simulink model "LPDs_single_agent_tech"  (R2023b)
settings: Solver=VariableStepAuto  StartTime=0.0  StopTime=24  FixedStep=0.005  RelTol=1e-6
undefined symbols (not defined in the file): battery_capacity_state_lower_limit, battery_capacity_state_upper_limit, battery_charge_power_state_lower_limit, battery_charge_power_state_upper_limit, battery_discharge_power_state_lower_limit, battery_discharge_power_state_upper_limit, battery_initial_capacity, battery_SOC_state_lower_limit, battery_SOC_state_upper_limit, EV_load_priority_factor, EV_load_rating, EV_load_state_lower_limit, EV_load_state_upper_limit, micro_grid_controller_power_state_lower_limit, micro_grid_controller_power_state_upper_limit, nano_grid_controller_power_rating, nano_grid_controller_power_state_lower_limit, nano_grid_controller_power_state_upper_limit, PV_power_rating, PV_power_state_lower_limit, PV_power_state_upper_limit, static_load_priority_factor, static_load_rating, static_load_state_lower_limit, static_load_state_upper_limit, sum_power_threshold_lower_limit, sum_power_threshold_upper_limit, TCL_load_priority_factor, TCL_load_rating, TCL_load_state_lower_limit, TCL_load_state_upper_limit, Wind_power_rating, Wind_power_state_lower_limit, Wind_power_state_upper_limit
libraries: spsStairGeneratorLib x13, simulink x7, slpidlib x2, rllib x2
(part 4 of 4)

== stateflow chart LPDs_single_agent_tech/Nano_Grid_Controller1/Chart ==
  settings: executeAtInitialization=1
  state Initialization1
    en:
    % Total Load
    %load = (static_load + TCL_load + EV_load)
  state Initialization2
    en:
    % Total Load
    load = (static_load + TCL_load + EV_load)
    % <------------------------------------------------------->
    % Nano Grid power parameters initiliazation
    % <------------------------------------------------------->
    nano_grid_supply = 0
    nano_grid_demand = 0
    %
    if Nano_grid_power < 0
    nano_grid_demand = abs(Nano_grid_power)
    else         % Nano_grid_power >= 0
    nano_grid_supply = Nano_grid_power
    end
    nano_grid_supply_out = nano_grid_supply
    nano_grid_demand_out = nano_grid_demand
    %
    nanogrid_usage = 0
    nanogrid_remain = nano_grid_supply
    %du:
    % <------------------------------------------------------->
    % Micro Grid power parameters initiliazation
    % <------------------------------------------------------->
    mg_power_usage_load = 0
    mg_power_usage_nanogrid = 0
    mg_power_usage = 0
  note: load_usage
      | source_power
      | error
      |
      |
      | PV_nanogrid_usage_percentage
      | nano_grid_supply_out
      | nano_grid_demand_mg_usage_percentage
      | nano_grid_demand_wind_usage_percentage
      | nano_grid_demand_wind_usage
      | nano_grid_demand_mg_usage
      | nanogrid_usage
      | nanogrid_remain
      | mg_power_usage
      | nano_grid_demand_out
  note: load_min > (PV + wind + battery + nanogrid)
  note: load > PV
  note: load > (PV + wind)
  note: load > (PV + wind + battery)
  state Use_Battery
    en:
    load_ = load - PV1_power - wind_power
  state load_flexibility
    en:
    load_ = load - PV1_power - wind_power - battery_discharging_power
    load_min = ksl_min*static_load + ktcl_min*TCL_load + kev_min*EV_load
    power_remain = PV1_power + wind_power + battery_discharging_power - load_min
  note: load_min > (PV + wind + battery)
  state Use_Wind
    en:
    load_ = load - PV1_power
  state use_nanogrid
    en:
    load_ = load_min - PV1_power - wind_power - battery_discharging_power
  state Use_microgrid
    en:
    load_ = load_min - PV1_power - wind_power - battery_discharging_power - nano_grid_supply
  state category_4
    en:
    source_power = PV1_power + wind_power + battery_discharging_power
    ks = ksl_min
    kt = ktcl_min
    ke = kev_min
    load = ks*static_load + kt*TCL_load + ke*EV_load
    error = source_power - load
    i = 0
    while (error > 1e-5) & (ks <= 1) & (kt <= 1) & (ke <= 1)
    if ks < 1
    ks = ks + 1e-5
    end
    if kt < 1
    kt = kt + 1e-5
    end
    if ke < 1
    ke = ke + 1e-5
    end
    load = ks*static_load + kt*TCL_load + ke*EV_load
    error = source_power - load
    i = i + 1
    end
  state category_1
    en:
    dPV = PV1_power - load
  state category_2
    en:
    dwind = PV1_power + wind_power - load
  state category_3
    en:
    dbattery = battery_discharging_power - load_
  state category_6
    en:
    Nano_grid_power_remain = PV1_power + wind_power + battery_discharging_power - load_min
    % Nano Grid power parameters
    nanogrid_usage =  load_min - PV1_power - wind_power - battery_discharging_power
  state category_7
    % Nano Grid power parameters
    nanogrid_usage =  nano_grid_supply
    en:
    mg_power_usage_load = load_
  state PV_Power_Mode_3
    % PV power parameters
    PV_load_usage = PV1_power
    % Wind power parameters
    wind_load_usage = wind_power
    % Battery power parameters
    battery_power = (PV1_power + wind_power) - load
    battery_charging_power_out = battery_power
    battery_discharging_power_out = 0
    battery_usage = battery_discharging_power_out
    % Load parameters
    static_load_usage = static_load
    TCL_load_usage = TCL_load
    EV_load_usage = EV_load
  state PV_Power_Mode_2
    % PV power parameters
    PV_load_usage = PV1_power
    % Wind power parameters
    wind_load_usage = load + battery_charging_power - PV1_power
    % Battery power parameters
    battery_charging_power_out = battery_charging_power
    battery_discharging_power_out = 0
    battery_usage = battery_discharging_power_out
    % Load parameters
    static_load_usage = static_load
    TCL_load_usage = TCL_load
    EV_load_usage = EV_load
  state PV_Power_Mode_1
    % PV power parameters
    PV_load_usage = load + battery_charging_power
    % Wind power parameters
    wind_load_usage = 0
    % Battery power parameters
    battery_charging_power_out = battery_charging_power
    battery_discharging_power_out = 0
    battery_usage = battery_discharging_power_out
    % Load parameters
    static_load_usage = static_load
    TCL_load_usage = TCL_load
    EV_load_usage = EV_load
  state PV_Wind_Power_Mode_2
    % PV power parameters
    PV_load_usage = PV1_power
    % Wind power parameters
    wind_load_usage = wind_power
    % Battery power parameters
    battery_power = PV1_power + wind_power - load
    battery_charging_power_out = battery_power
    battery_discharging_power_out = 0
    battery_usage = battery_discharging_power_out
    % Load parameters
    static_load_usage = static_load
    TCL_load_usage = TCL_load
    EV_load_usage = EV_load
  state PV_Wind_Battery_Power_Mode
    % PV power parameters
    PV_load_usage = PV1_power
    % Wind power parameters
    wind_load_usage = wind_power
    % Battery power parameters
    battery_power =  load - PV1_power - wind_power
    battery_charging_power_out = 0
    battery_discharging_power_out = battery_power
    battery_usage = battery_discharging_power_out
    % Load parameters
    static_load_usage = static_load
    TCL_load_usage = TCL_load
    EV_load_usage = EV_load
  state PV_Wind_Power_Mode_1
    % PV power parameters
    PV_load_usage = PV1_power
    % Wind power parameters
    wind_load_usage = load + battery_charging_power - PV1_power
    % Battery power parameters
    battery_charging_power_out = battery_charging_power
    battery_discharging_power_out = 0
    battery_usage = battery_discharging_power_out
    % Load parameters
    static_load_usage = static_load
    TCL_load_usage = TCL_load
    EV_load_usage = EV_load
  state PV_Wind_Battery_Power_Mode_load_min1
    % PV power parameters
    PV_load_usage = PV1_power
    % Wind power parameters
    wind_load_usage = wind_power
    % Battery power parameters
    battery_charging_power_out = 0
    battery_discharging_power_out = battery_discharging_power
    battery_usage = battery_discharging_power_out
    % Load parameters
    static_load_usage = ksl_min*static_load
    TCL_load_usage = ktcl_min*TCL_load
    EV_load_usage = kev_min*EV_load
    % Nano Grid power parameters
    nanogrid_remain = nano_grid_supply - nanogrid_usage
  state PV_Wind_Battery_Power_Mode_load_min
    % PV power parameters
    PV_load_usage = PV1_power
    % Wind power parameters
    wind_load_usage = wind_power
    % Battery power parameters
    battery_power =  load - PV1_power - wind_power
    battery_charging_power_out = 0
    battery_discharging_power_out = battery_discharging_power
    battery_usage = battery_discharging_power_out
    % Load parameters
    static_load_usage = ks*static_load
    TCL_load_usage = kt*TCL_load
    EV_load_usage = ke*EV_load
  state Nano_Grid_Initiliazation
    %
    nano_grid_demand_PV_usage = 0
    nano_grid_demand_wind_usage = 0
    nano_grid_demand_mg_usage = 0
    PV_nanogrid_usage = 0
    wind_nanogrid_usage = 0
    %
    PV_remain = PV1_power - PV_load_usage
    wind_remain = wind_power - wind_load_usage
    %
    PV_remain_ = PV_remain
    wind_remain_ = wind_remain
    Remain_source_power = PV_remain + wind_remain
  note: 0 < nano_grid_demand < PV_remain
  state ds
    nano_grid_demand_PV_usage = nano_grid_demand
  state el
    dP = PV_remain - nano_grid_demand
  note: nano_grid_demand > PV_remain
  note: (PV_remain) < nano_grid_demand < (PV_remain + wind_remain)
  state ell
    nano_grid_demand_PV_usage = PV_remain
    dPw = PV_remain + wind_remain - nano_grid_demand
  state ds1
    nano_grid_demand_wind_usage = nano_grid_demand - nano_grid_demand_PV_usage
  note: nano_grid_demand > PV_remain + wind_remain
  state ell1
    nano_grid_demand_wind_usage = wind_remain
    mg = nano_grid_demand - nano_grid_demand_PV_usage - nano_grid_demand_wind_usage
    nano_grid_demand_mg_usage = mg
    mg_power_usage_nanogrid = mg
    %
    Remain_source_power = 0
  state fi
    PV_remain_ = PV_remain - nano_grid_demand_PV_usage
    wind_remain_ = wind_remain - nano_grid_demand_wind_usage
    %
    PV_nanogrid_usage = nano_grid_demand_PV_usage
    wind_nanogrid_usage = nano_grid_demand_wind_usage
    %
    Remain_source_power = PV_remain_ + wind_remain_
  state PV %  battery_charging_power =< PV_remain
    en:
    % PV Power Parameters
    PV_load_usage_percentage = 100*PV_load_usage/PV1_power
    PV_nanogrid_usage_percentage = 100*nano_grid_demand_PV_usage/PV1_power
    PV_remain_percentage = 100*PV_remain_/PV1_power
    % Wind Power Parameters
    wind_load_usage_percentage = 100*wind_load_usage/wind_power
    wind_nanogrid_usage_percentage = 100*nano_grid_demand_wind_usage/wind_power
    wind_remain_percentage = 100*wind_remain_/wind_power
    % Battery Charging Power Parameters
    a = 100*battery_charging_power_out/battery_charging_power
    battery_charging_power_out_percentage = a
    % Battery Discharging Power Parameters
    b = 100*battery_discharging_power_out/battery_discharging_power
    battery_discharging_power_out_percentage = b
    % Static Load
    static_load_usage_percentage = 100*static_load_usage/static_load
    % TCL Load
    TCL_load_usage_percentage = 100*TCL_load_usage/TCL_load
    % EV Load
    EV_load_usage_percentage = 100*EV_load_usage/EV_load
    load_usage = static_load_usage + TCL_load_usage + EV_load_usage
    % Nano Grid
    nano_grid_demand_PV_usage_percentage = 100*nano_grid_demand_PV_usage/nano_grid_demand
    nano_grid_demand_wind_usage_percentage = 100*nano_grid_demand_wind_usage/nano_grid_demand
    nano_grid_demand_mg_usage_percentage = 100*nano_grid_demand_mg_usage/nano_grid_demand
    % Micro Grid
    mg_power_usage = mg_power_usage_nanogrid + mg_power_usage_load
    % Power balance check
    total_power_produced = PV1_power + wind_power + battery_discharging_power + nano_grid_supply + mg_power_usage
    total_power_consumed = static_load_usage + TCL_load_usage + EV_load_usage + battery_charging_power_out + nano_grid_demand
    power_balance_error = total_power_produced - total_power_consumed
  state Output_parameters
    en:
    % PV_param
    PV_param = [PV1_power PV_load_usage PV_nanogrid_usage PV_remain_...
    PV_load_usage_percentage PV_nanogrid_usage_percentage PV_remain_percentage]
    % wind_param
    wind_param = [wind_power wind_load_usage wind_nanogrid_usage wind_remain_...
    wind_load_usage_percentage wind_nanogrid_usage_percentage wind_remain_percentage]
    % battery_charging_param
    battery_charging_param =      [battery_charging_power     battery_charging_power_out      battery_charging_power_out_percentage]
    battery_discharging_param = [battery_discharging_power battery_discharging_power_out battery_discharging_power_out_percentage battery_usage]
    % Load param
    static_load_param =  [static_load static_load_usage static_load_usage_percentage]
    TCL_load_param =  [TCL_load TCL_load_usage TCL_load_usage_percentage]
    EV_load_param =  [EV_load EV_load_usage EV_load_usage_percentage]
    % nanogrid param
    nano_grid_supply_param = [nano_grid_supply nanogrid_usage nanogrid_remain]
    nano_grid_demand_param = [nano_grid_demand nano_grid_demand_PV_usage nano_grid_demand_PV_usage_percentage...
    nano_grid_demand_wind_usage nano_grid_demand_wind_usage_percentage nano_grid_demand_mg_usage...
    nano_grid_demand_mg_usage_percentage]
    % microgrid param
    mg_param = [micro_grid_power mg_power_usage mg_power_usage_load mg_power_usage_nanogrid]
    % power balance
    power_production = [PV1_power wind_power battery_discharging_power nano_grid_supply mg_power_usage]
    power_consumption = [static_load_usage TCL_load_usage EV_load_usage battery_charging_power_out nano_grid_demand]
    load_source_balance = [total_power_produced total_power_consumed power_balance_error]
    %PVVV = PV1_power
  (default) -> Initialization1
  Initialization1 -> Initialization2
  Initialization2 -> (junction 488)
  Use_Wind -> Use_Battery [order 2] : [load > wind_power]
  (junction 488) -> Use_Wind [order 2]
  Use_Battery -> load_flexibility [order 2]
  use_nanogrid -> Use_microgrid [order 2]
  (junction 488) -> category_1 [order 1] : [load <= PV1_power]
  load_flexibility -> use_nanogrid [order 2]
  Use_Wind -> category_2 [order 1] : [load_ <= wind_power]
  Use_Battery -> category_3 [order 1] : [load_ <= battery_discharging_power]
  use_nanogrid -> category_6 [order 1] : [load_ <= nano_grid_supply]
  Use_microgrid -> category_7
  load_flexibility -> category_4 [order 1] : [power_remain >= 0]
  category_1 -> PV_Power_Mode_3 [order 3]
  category_1 -> PV_Power_Mode_1 [order 1] : [dPV >= battery_charging_power]
  category_3 -> PV_Wind_Battery_Power_Mode
  category_1 -> PV_Power_Mode_2 [order 2] : [(dPV + wind_power) >= battery_charging_power]
  category_2 -> PV_Wind_Power_Mode_1 [order 1] : [dwind >= battery_charging_power]
  category_2 -> PV_Wind_Power_Mode_2 [order 2]
  category_7 -> PV_Wind_Battery_Power_Mode_load_min1
  category_6 -> PV_Wind_Battery_Power_Mode_load_min1
  category_4 -> PV_Wind_Battery_Power_Mode_load_min
  PV_Power_Mode_2 -> Nano_Grid_Initiliazation
  PV_Power_Mode_1 -> Nano_Grid_Initiliazation
  PV_Wind_Power_Mode_1 -> Nano_Grid_Initiliazation
  PV_Power_Mode_3 -> Nano_Grid_Initiliazation
  PV_Wind_Power_Mode_2 -> Nano_Grid_Initiliazation
  PV_Wind_Battery_Power_Mode -> Nano_Grid_Initiliazation
  PV_Wind_Battery_Power_Mode_load_min1 -> Nano_Grid_Initiliazation
  PV_Wind_Battery_Power_Mode_load_min -> Nano_Grid_Initiliazation
  Nano_Grid_Initiliazation -> PV %  battery_charging_power =< PV_remain [order 2]
  Nano_Grid_Initiliazation -> el [order 1] : [nano_grid_demand > 0]
  el -> ds [order 2]
  ds -> fi
  el -> ell [order 1] : [dP < 0]
  ell -> ds1 [order 2]
  ell -> ell1 [order 1] : [dPw < 0]
  ds1 -> fi
  ell1 -> fi
  fi -> PV %  battery_charging_power =< PV_remain
  PV %  battery_charging_power =< PV_remain -> Output_parameters
  data: Nano_grid_power input; static_load input; TCL_load input; EV_load input; micro_grid_power input; wind_power input; load_ local; a local; b local; kev_min constant double =EV_load_priority_factor; ktcl_min constant double =TCL_load_priority_factor; power_remain local; load_min local; ksl_min constant double =static_load_priority_factor; ks local; i local; ke local; kt local; dwind local; dPV local; battery_power local; dbattery local; Nano_grid_power_remain local; battery_discharging_power input; load local; nano_grid_demand local; nano_grid_supply local; mg_power_usage_nanogrid local; PV_remain local; wind_remain local; mg_power_usage_load local; Remain_source_power local; dPw local; dP local; mg local; PV_param output; nano_grid_demand_PV_usage local; PV_load_usage local; nano_grid_demand_PV_usage_percentage local; PV_load_usage_percentage local; PV_remain_ local; wind_param output; wind_nanogrid_usage_percentage local; wind_load_usage_percentage local; wind_remain_ local; wind_load_usage local; battery_discharging_param output; battery_charging_param output; battery_charging_power input; battery_charging_power_out local; battery_charging_power_out_percentage local; battery_discharging_power_out local; battery_discharging_power_out_percentage local; battery_usage local; static_load_param output; static_load_usage local; static_load_usage_percentage local; TCL_load_param output; TCL_load_usage_percentage local; TCL_load_usage local; EV_load_param output; EV_load_usage_percentage local; EV_load_usage local; nano_grid_demand_param output; nano_grid_supply_param output; mg_param output; mg_power_usage local; nano_grid_demand_mg_usage local; nano_grid_demand_mg_usage_percentage local; nano_grid_demand_out local; nano_grid_demand_wind_usage local; nano_grid_demand_wind_usage_percentage local; nano_grid_supply_out local; nanogrid_remain local; nanogrid_usage local; load_source_balance output; load_usage local; source_power local; error local; PV_nanogrid_usage_percentage local; PV1_power input; PV_nanogrid_usage local; wind_nanogrid_usage local; wind_remain_percentage local; PV_remain_percentage local; power_balance_error local; total_power_produced local; total_power_consumed local; power_consumption output; power_production output

== stateflow chart LPDs_single_agent_tech/BESS_10 kWh/BESSs, battery SOC ------ > charging, discharging. power ==
  settings: executeAtInitialization=1
  state state
  state Battery_SOC_max
    %batteryState = MAX
    battery_charge_factor = charge_min
    battery_discharge_factor = discharge_max
  state BatteryHigh
    %batteryState = HIGH;
    battery_charge_factor = charge_low
    battery_discharge_factor = discharge_high
  state Normal
    %batteryState = NORMAL;
    battery_charge_factor = charge_medium;
    battery_discharge_factor = discharge_medium;
  state Battery_SOC_max1
    %batteryState = MAX
    battery_charging_power = battery_charge_factor*battery_charging_power_upper_limits
    battery_discharging_power = battery_discharge_factor*battery_discharging_power_upper_limits
  state BatteryLow
    %batteryState = LOW;
    battery_charge_factor = charge_high;
    battery_discharge_factor = discharge_low;
  state BatteryMin
    %batteryState = MIN;
    battery_charge_factor = charge_max
    battery_discharge_factor = discharge_min
  (default) -> state
  state -> (junction 261)
  (junction 261) -> Battery_SOC_max [order 1] : [battery_SOC >= SOC_max]
  Battery_SOC_max -> Battery_SOC_max1
  (junction 261) -> (junction 243) [order 2]
  BatteryHigh -> Battery_SOC_max1
  (junction 243) -> BatteryHigh [order 1] : [battery_SOC >= SOC_high]
  (junction 243) -> (junction 257) [order 2]
  (junction 257) -> Normal [order 1] : [battery_SOC >= SOC_low]
  Normal -> Battery_SOC_max1
  (junction 257) -> (junction 269) [order 2]
  BatteryLow -> Battery_SOC_max1
  BatteryMin -> Battery_SOC_max1
  (junction 269) -> BatteryLow [order 1] : [battery_SOC >= SOC_min]
  (junction 269) -> (junction 249) [order 2]
  (junction 249) -> BatteryMin
  data: battery_SOC input; battery_SOC_upper_limits input; battery_SOC_lower_limits input; SOC_high constant double =0.80; SOC_low constant double =0.30; SOC_min constant double =0.15; SOC_max constant double =0.95; charge_max local =1; charge_high local =0.95; charge_medium local =0.8; charge_low local =0.5; charge_min local =0.2; discharge_min local =0; discharge_low local =0.1; discharge_medium local =0.8; discharge_high local =0.95; discharge_max local =1; battery_charge_factor output; battery_discharge_factor output; HIGH local; LOW local; MAX local; MIN local; NORMAL local; battery_charging_power output; battery_discharging_power output; battery_charging_power_upper_limits input; battery_discharging_power_upper_limits input; batteryState local

== matlab function LPDs_single_agent_tech/Nano_Grid_Controller1/MATLAB Function ==
  data: u input; y output
function y = f(u)

%% Argument extraction
PV1_power = u(1);
wind_power = u(2);
battery_discharging_power = u(3);
battery_charging_power = u(4);
micro_grid_power = u(5);
Nano_grid_power = u(6);
static_load = u(7);
TCL_load = u(8);
EV_load = u(9);
static_load_priority_factor = u(10);
TCL_load_priority_factor = u(11);
EV_load_priority_factor = u(12);

%%
ksl_min = static_load_priority_factor;
ktcl_min = TCL_load_priority_factor;
kev_min = EV_load_priority_factor;
error = NaN;
%% Initialization 2
% Total Load
load = (static_load + TCL_load + EV_load);
load_min = ksl_min*static_load + ktcl_min*TCL_load + kev_min*EV_load;
% <------------------------------------------------------->
% Nano Grid power parameters initiliazation
% <------------------------------------------------------->
nano_grid_supply = 0;
nano_grid_demand = 0;
%
if Nano_grid_power < 0
   nano_grid_demand = abs(Nano_grid_power);
else         % Nano_grid_power >= 0
   nano_grid_supply = Nano_grid_power;
end
nano_grid_supply_out = nano_grid_supply;
nano_grid_demand_out = nano_grid_demand;
%
nanogrid_usage = 0;
nanogrid_remain = nano_grid_supply;
% <------------------------------------------------------->
% Micro Grid power parameters initiliazation
% <------------------------------------------------------->
mg_power_usage_load = 0;
mg_power_usage_nanogrid = 0;
mg_power_usage = 0;


%% Use PV, load < PV
if load <= PV1_power
   %% category_1
   dPV = PV1_power - load;
   if dPV >= battery_charging_power
      % PV_Power_Mode_1
      % PV power parameters
      PV_load_usage = load + battery_charging_power;
      % Wind power parameters
      wind_load_usage = 0;
      % Battery power parameters
      battery_charging_power_out = battery_charging_power;
      battery_discharging_power_out = 0;
      battery_usage = battery_discharging_power_out;
      % Load parameters
      static_load_usage = static_load;
      TCL_load_usage = TCL_load;
      EV_load_usage = EV_load;

   elseif (dPV + wind_power) >= battery_charging_power
      % PV_Power_Mode_2
      % PV power parameters
      PV_load_usage = PV1_power;
      % Wind power parameters
      wind_load_usage = load + battery_charging_power - PV1_power;
      % Battery power parameters
      battery_charging_power_out = battery_charging_power;
      battery_discharging_power_out = 0;
      battery_usage = battery_discharging_power_out;
      % Load parameters
      static_load_usage = static_load;
      TCL_load_usage = TCL_load;
      EV_load_usage = EV_load;

   else
      % PV_Power_Mode_3
      % PV power parameters
      PV_load_usage = PV1_power;
      % Wind power parameters
      wind_load_usage = wind_power;
      % Battery power parameters
      battery_power = (PV1_power + wind_power) - load;
      battery_charging_power_out = battery_power;
      battery_discharging_power_out = 0;
      battery_usage = battery_discharging_power_out;
      % Load parameters
      static_load_usage = static_load;
      TCL_load_usage = TCL_load;
      EV_load_usage = EV_load;
   end



   %% Use_Wind
elseif load <= (PV1_power + wind_power)
   % category_2
   dwind = PV1_power + wind_power - load;
   if dwind >= battery_charging_power
      % PV_Wind_Power_Mode_1
      % PV power parameters
      PV_load_usage = PV1_power;
      % Wind power parameters
      wind_load_usage = load + battery_charging_power - PV1_power;
      % Battery power parameters
      battery_charging_power_out = battery_charging_power;
      battery_discharging_power_out = 0;
      battery_usage = battery_discharging_power_out;
      % Load parameters
      static_load_usage = static_load;
      TCL_load_usage = TCL_load;
      EV_load_usage = EV_load;
   else
      % PV_Wind_Power_Mode_2
      % PV power parameters
      PV_load_usage = PV1_power;
      % Wind power parameters
      wind_load_usage = wind_power;
      % Battery power parameters
      battery_power = PV1_power + wind_power - load;
      battery_charging_power_out = battery_power;
      battery_discharging_power_out = 0;
      battery_usage = battery_discharging_power_out;
      % Load parameters
      static_load_usage = static_load;
      TCL_load_usage = TCL_load;
      EV_load_usage = EV_load;
   end



   %% Use Battery
elseif load <= (PV1_power + wind_power + battery_discharging_power)
   %category_3
   dbattery = PV1_power + wind_power + battery_discharging_power - load;
   % PV_Wind_Battery_Power_Mode
   % PV power parameters
   PV_load_usage = PV1_power;
   % Wind power parameters
   wind_load_usage = wind_power;
   % Battery power parameters
   battery_power =  load - PV1_power - wind_power;
   battery_charging_power_out = 0;
   battery_discharging_power_out = battery_power;
   battery_usage = battery_discharging_power_out;
   % Load parameters
   static_load_usage = static_load;
   TCL_load_usage = TCL_load;
   EV_load_usage = EV_load;


   
   %% Flexibilized Load
elseif load_min <= (PV1_power + wind_power + battery_discharging_power)
   % category_4 
   source_power = PV1_power + wind_power + battery_discharging_power;
   ks = ksl_min;
   kt = ktcl_min;
   ke = kev_min;
   load = ks*static_load + kt*TCL_load + ke*EV_load;
   error = source_power - load;
   i = 0;
   while (error > 1e-5) && (ks <= 1) && (kt <= 1) && (ke <= 1)
      if ks < 1
          ks = ks + 1e-5;
      end
      if kt < 1
          kt = kt + 1e-5;
      end
      if ke < 1
          ke = ke + 1e-5;
      end
      load = ks*static_load + kt*TCL_load + ke*EV_load;
      error = source_power - load;
      i = i + 1;
   end
   % PV_Wind_Battery_Power_Mode_load_min
   % PV power parameters
   PV_load_usage = PV1_power;
   % Wind power parameters
   wind_load_usage = wind_power;
   % Battery power parameters
   battery_power =  load - PV1_power - wind_power;
   battery_charging_power_out = 0;
   battery_discharging_power_out = battery_discharging_power;
   battery_usage = battery_discharging_power_out;
   % Load parameters
   static_load_usage = ks*static_load;
   TCL_load_usage = kt*TCL_load;
   EV_load_usage = ke*EV_load;



   %% use nanogrid and minimize load
elseif load_min <= (PV1_power + wind_power + battery_discharging_power + nano_grid_supply)
   % category_6
   Nano_grid_power_remain = PV1_power + wind_power + battery_discharging_power - load_min;
   % Nano Grid power parameters
   nanogrid_usage =  load_min - PV1_power - wind_power - battery_discharging_power;

   % PV_Wind_Battery_Power_Mode_load_min1
   % PV power parameters
   PV_load_usage = PV1_power;
   % Wind power parameters
   wind_load_usage = wind_power;
   % Battery power parameters
   battery_charging_power_out = 0;
   battery_discharging_power_out = battery_discharging_power;
   battery_usage = battery_discharging_power_out;
   % Load parameters
   static_load_usage = ksl_min*static_load;
   TCL_load_usage = ktcl_min*TCL_load;
   EV_load_usage = kev_min*EV_load;
   % Nano Grid power parameters
   nanogrid_remain = nano_grid_supply - nanogrid_usage;


   
   %% Use Microgrid
else
   % Use_microgrid
   load_ = load_min - PV1_power - wind_power - battery_discharging_power - nano_grid_supply;
   % category_7
   % Nano Grid power parameters
   nanogrid_usage =  nano_grid_supply;
   mg_power_usage_load = load_;
   
   % PV_Wind_Battery_Power_Mode_load_min1
   % PV power parameters
   PV_load_usage = PV1_power;
   % Wind power parameters
   wind_load_usage = wind_power;
   % Battery power parameters
   battery_charging_power_out = 0;
   battery_discharging_power_out = battery_discharging_power;
   battery_usage = battery_discharging_power_out;
   % Load parameters
   static_load_usage = ksl_min*static_load;
   TCL_load_usage = ktcl_min*TCL_load;
   EV_load_usage = kev_min*EV_load;
   % Nano Grid power parameters
   nanogrid_remain = nano_grid_supply - nanogrid_usage;
end


%% Nano_Grid_Initialization
%
nano_grid_demand_PV_usage = 0;
nano_grid_demand_wind_usage = 0;
nano_grid_demand_mg_usage = 0;
PV_nanogrid_usage = 0;
wind_nanogrid_usage = 0;
%
PV_remain = PV1_power - PV_load_usage;
wind_remain = wind_power - wind_load_usage;
%
PV_remain_ = PV_remain;
wind_remain_ = wind_remain;
Remain_source_power = PV_remain + wind_remain;

%%
if nano_grid_demand >= 0
   dP = PV_remain - nano_grid_demand;
   if dP > 0
       nano_grid_demand_PV_usage = nano_grid_demand;
   else   %  dP < 0
       nano_grid_demand_PV_usage = PV_remain;
       dPw = PV_remain + wind_remain - nano_grid_demand;
       if dPw >= 0
           nano_grid_demand_wind_usage = nano_grid_demand - nano_grid_demand_PV_usage;
       else % dPw < 0
           nano_grid_demand_wind_usage = wind_remain;
           mg = nano_grid_demand - nano_grid_demand_PV_usage - nano_grid_demand_wind_usage;
           nano_grid_demand_mg_usage = mg;
           mg_power_usage_nanogrid = mg;
           %
           Remain_source_power = 0;
       end
   end

   PV_remain_ = PV_remain - nano_grid_demand_PV_usage;
   wind_remain_ = wind_remain - nano_grid_demand_wind_usage;
   %
   PV_nanogrid_usage = nano_grid_demand_PV_usage;
   wind_nanogrid_usage = nano_grid_demand_wind_usage;
   %
   Remain_source_power = PV_remain_ + wind_remain_;
end

% PV %  battery_charging_power =< PV_remain

% PV Power Parameters
PV_load_usage_percentage = 100*PV_load_usage/PV1_power;
PV_nanogrid_usage_percentage = 100*nano_grid_demand_PV_usage/PV1_power;
PV_remain_percentage = 100*PV_remain_/PV1_power;
% Wind Power Parameters
wind_load_usage_percentage = 100*wind_load_usage/wind_power;
wind_nanogrid_usage_percentage = 100*nano_grid_demand_wind_usage/wind_power;
wind_remain_percentage = 100*wind_remain_/wind_power;
% Battery Charging Power Parameters
a = 100*battery_charging_power_out/battery_charging_power;
battery_charging_power_out_percentage = a;
% Battery Discharging Power Parameters
b = 100*battery_discharging_power_out/battery_discharging_power;
battery_discharging_power_out_percentage = b;
% Static Load
static_load_usage_percentage = 100*static_load_usage/static_load;
% TCL Load
TCL_load_usage_percentage = 100*TCL_load_usage/TCL_load;
% EV Load
EV_load_usage_percentage = 100*EV_load_usage/EV_load;
load_usage = static_load_usage + TCL_load_usage + EV_load_usage;
% Nano Grid
nano_grid_demand_PV_usage_percentage = 100*nano_grid_demand_PV_usage/nano_grid_demand;
nano_grid_demand_wind_usage_percentage = 100*nano_grid_demand_wind_usage/nano_grid_demand;
nano_grid_demand_mg_usage_percentage = 100*nano_grid_demand_mg_usage/nano_grid_demand;
% Micro Grid
mg_power_usage = mg_power_usage_nanogrid + mg_power_usage_load;
% Power balance check
total_power_produced = PV1_power + wind_power + battery_discharging_power + nano_grid_supply + mg_power_usage;
total_power_consumed = static_load_usage + TCL_load_usage + EV_load_usage + battery_charging_power_out + nano_grid_demand;
power_balance_error = total_power_produced - total_power_consumed;



%% Output_parameters
% PV_param
PV_param = [PV1_power PV_load_usage PV_nanogrid_usage PV_remain_ PV_load_usage_percentage PV_nanogrid_usage_percentage PV_remain_percentage];
% wind_param
wind_param = [wind_power wind_load_usage wind_nanogrid_usage wind_remain_ wind_load_usage_percentage wind_nanogrid_usage_percentage wind_remain_percentage];
% battery_charging_param
battery_charging_param =      [battery_charging_power     battery_charging_power_out      battery_charging_power_out_percentage];
battery_discharging_param = [battery_discharging_power battery_discharging_power_out battery_discharging_power_out_percentage battery_usage];
% Load param
static_load_param =  [static_load static_load_usage static_load_usage_percentage];
TCL_load_param =  [TCL_load TCL_load_usage TCL_load_usage_percentage];
EV_load_param =  [EV_load EV_load_usage EV_load_usage_percentage];
% nanogrid param
nano_grid_supply_param = [nano_grid_supply nanogrid_usage nanogrid_remain];
nano_grid_demand_param = [nano_grid_demand nano_grid_demand_PV_usage nano_grid_demand_PV_usage_percentage...
   nano_grid_demand_wind_usage nano_grid_demand_wind_usage_percentage nano_grid_demand_mg_usage...
   nano_grid_demand_mg_usage_percentage];
% microgrid param
mg_param = [micro_grid_power mg_power_usage mg_power_usage_load mg_power_usage_nanogrid];
% power balance
power_production = [PV1_power wind_power battery_discharging_power nano_grid_supply mg_power_usage];
power_consumption = [static_load_usage TCL_load_usage EV_load_usage battery_charging_power_out nano_grid_demand];
load_source_balance = [total_power_produced total_power_consumed power_balance_error];

%% 
y = [PV_param wind_param battery_charging_param battery_discharging_param static_load_param TCL_load_param EV_load_param nano_grid_supply_param nano_grid_demand_param...
     mg_param load_source_balance power_production power_consumption error];
